simulink model "apogeeManeuver"  (R2023a)
settings: Solver=ode4  StartTime=0.0  StopTime=10.0  FixedStep=dt  RelTol=1e-3
libraries: simulink x1
settings Model: Creator=ndelurgio  LastModifiedBy=ndelurgio

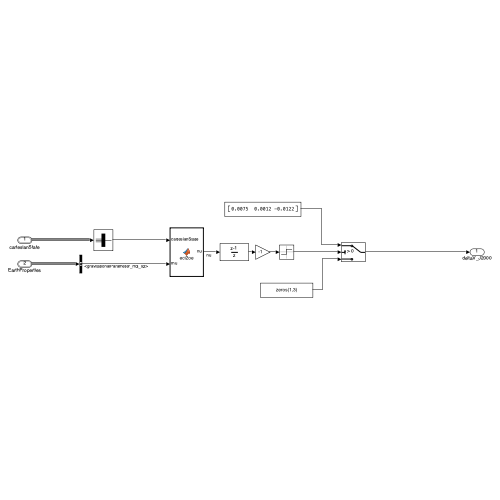
[thumbnail: Simulink's stored preview of the top-level diagram]
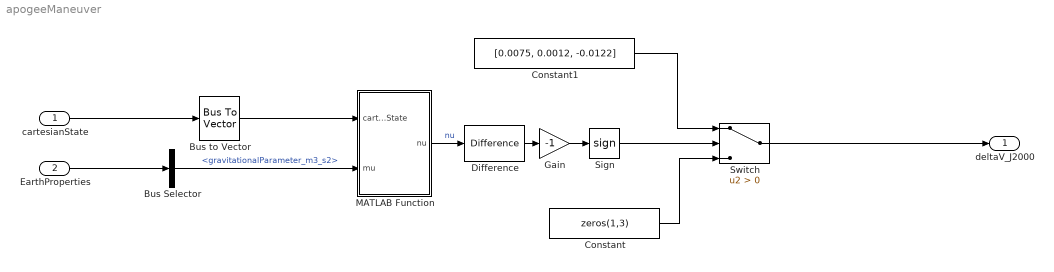
== system apogeeManeuver ==
  cartesianState : Inport  OutDataTypeStr=Bus: cartesianState
  EarthProperties : Inport  Port=2  OutDataTypeStr=Bus: earthProperties
  Bus Selector : BusSelector  OutputSignals=gravitationalParameter_m3_s2
  Bus to Vector : BusToVector
  Constant : Constant  Value=zeros(1,3)
  Constant1 : Constant  Value=[0.0075, 0.0012, -0.0122]
  Difference : simulink/Discrete/Difference  ICPrevInput=0.0  OutMin=[]  OutMax=[]  OutDataType=fixdt(1, 16)  OutScaling=2^-10  DoSatur=off
  Gain : Gain  Gain=-1
  MATLAB Function : MATLAB Function  TreatAsAtomicUnit=on
  Sign : Signum
  Switch : Switch  Criteria=u2 > Threshold  SaturateOnIntegerOverflow=off  InputSameDT=off
  deltaV_J2000 : Outport
  wires:
  cartesianState/1 -> Bus to Vector/1
  Bus to Vector/1 -> MATLAB Function/1(cartesianState)
  EarthProperties/1 -> Bus Selector/1
  Bus Selector/1 -> MATLAB Function/2(mu)  "<gravitationalParameter_m3_s2>"
  MATLAB Function/1(nu) -> Difference/1  "nu"
  Sign/1 -> Switch/2
  Difference/1 -> Gain/1
  Gain/1 -> Sign/1
  Constant/1 -> Switch/3
  Constant1/1 -> Switch/1
  Switch/1 -> deltaV_J2000/1

== matlab function apogeeManeuver/MATLAB Function ==
  data: cartesianState input; nu output; mu input
function nu = eci2oe(cartesianState,mu)
oe = eci2oe(cartesianState,mu);
nu = oe(6);
end
